simulink model "c28x_spi_eeprom"  (R2021b)
settings: Solver=FixedStepDiscrete  StartTime=0.0  StopTime=Inf  FixedStep=0.001  RelTol=1e-3  EnableMultiTasking=on
libraries: c280xlib x4, svdutilitieslib x2, simulink x2, demo_controls x1
settings Model: SimulationMode=external  ExtModeTrigDuration=8  Creator=The MathWorks, Inc.  LastModifiedBy=The MathWorks, Inc.
settings SolverCC: AlgebraicLoopSolver=TrustRegion
settings DataIOCC: ReturnWorkspaceOutputs=off
settings OptimizationCC: DefaultUnderspecifiedDataType=single  EnhancedBackFolding=on  StrengthReduction=on  PassReuseOutputArgsAs=Individual arguments  MaxStackSize=512  OptimizeBlockOrder=speed  DifferentSizesBufferReuse=on  EfficientTunableParamExpr=on
settings DebuggingCC: InheritedTsInSrcMsg=none  ParameterPrecisionLossMsg=none  ParameterTunabilityLossMsg=error  SFMachineParentedDataDiag=warning  ArithmeticOperatorsInVariantConditions=warning
settings HardwareCC: ProdBitPerChar=16  ProdBitPerInt=16  ProdBitPerPointer=32  ProdBitPerSizeT=32  ProdBitPerPtrDiffT=32  ProdLargestAtomicInteger=Integer  ProdLargestAtomicFloat=None  ProdWordSize=16  ProdLongLongMode=on  ProdHWDeviceType=Texas Instruments->C2000
settings SFSimCC: SimUseLocalCustomCode=off  MATLABDynamicMemAlloc=off  CustomCodeUndefinedFunction=UseInterfaceOnly
settings RTWCC: Description=Embedded Coder  SystemTargetFile=ert.tlc  HardwareBoard=TI Delfino F28379D LaunchPad  TemplateMakefile=ert_default_tmf  GenerateReport=on  RTWUseLocalCustomCode=off  Toolchain=Texas Instruments Code Composer Studio (C2000)  IncludeHyperlinkInReport=on  LaunchReport=on  GenerateTraceInfo=on  GenerateTraceReport=on  GenerateTraceReportSl=on  GenerateTraceReportSf=on  GenerateTraceReportEml=on
settings CodeAppCC: ForceParamTrailComments=on  IgnoreCustomStorageClasses=off  OperatorAnnotations=on  SimulinkDataObjDesc=on  SFDataObjDesc=on  InsertBlockDesc=on
settings ERTTargetCC: CodeReplacementLibrary=TI C28x  ExtModeTransport=4  ExtModeStaticAlloc=on  ExtModeStaticAllocSize=10000  ExtModeMexFile=ext_xcp  ExtModeIntrfLevel=Level2 - Open

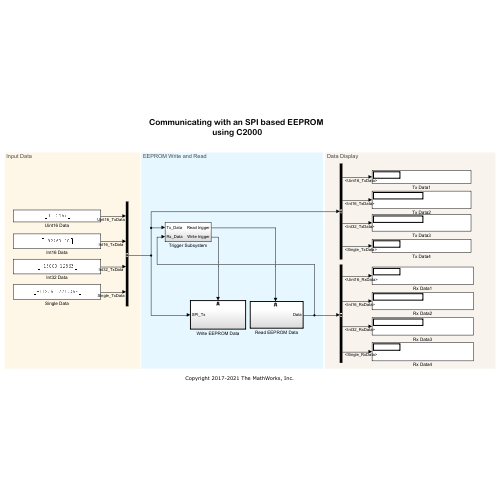
[thumbnail: Simulink's stored preview of the top-level diagram]
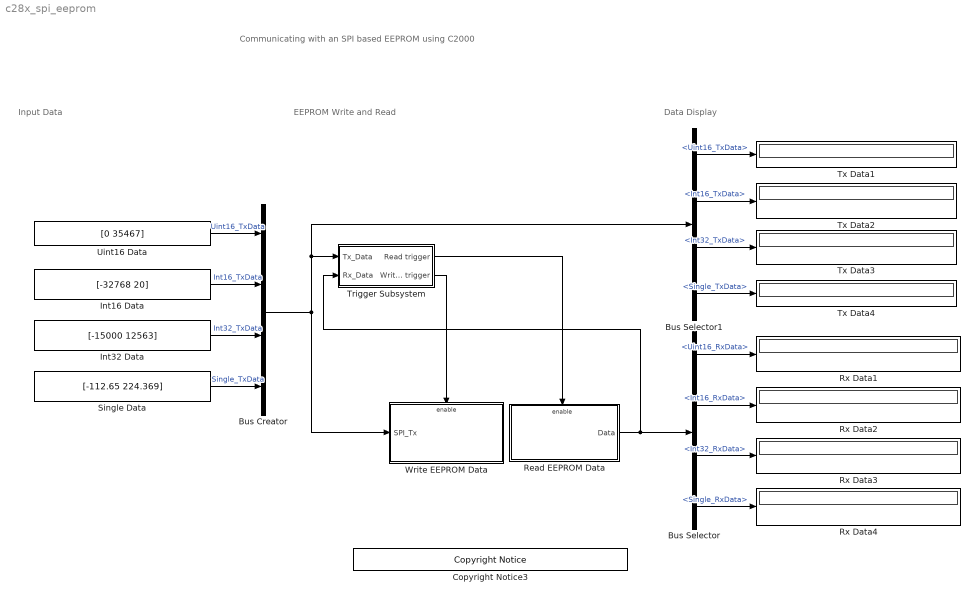
== system c28x_spi_eeprom ==
  note: Communicating with an SPI based EEPROM
      | using C2000
  note: Input Data
  note: EEPROM Write and Read
  note: Data Display
  Bus Creator : BusCreator  Inputs=4
  Bus Selector : BusSelector  OutputSignals=Uint16_RxData,Int16_RxData,Int32_RxData,Single_RxData
  Bus Selector1 : BusSelector  OutputSignals=Uint16_TxData,Int16_TxData,Int32_TxData,Single_TxData
  Copyright Notice3 : demo_controls/Copyright Notice  year=2017  prod=tic2000
      settings: SourceProductBaseCode=ME
  Int16 Data : Constant  Value=[-32768 20]  OutDataTypeStr=int16  SampleTime=-1
  Int32 Data : Constant  Value=[-15000 12563]  OutDataTypeStr=int32  SampleTime=-1
  Read EEPROM Data : Subsystem  TreatAsAtomicUnit=on
  Rx Data{1..4} (4 alike) : Display
      Rx Data4 settings: Format=short_e
  Single Data : Constant  Value=[-112.65 224.369]  OutDataTypeStr=single  SampleTime=-1
  Trigger Subsystem : Subsystem
  Tx Data{1..4} (4 alike) : Display
      Tx Data4 settings: Format=short_e
  Uint16 Data : Constant  Value=[0 35467]  OutDataTypeStr=uint16  SampleTime=-1
  Write EEPROM Data : Subsystem
  wires:
  Trigger Subsystem/1(Read trigger) -> Read EEPROM Data/Enable
  Bus Creator/1 -> Bus Selector1/1, Trigger Subsystem/1(Tx_Data), Write EEPROM Data/1(SPI_Tx)
  Read EEPROM Data/1(Data) -> Trigger Subsystem/2(Rx_Data), Bus Selector/1
  Trigger Subsystem/2(Write trigger) -> Write EEPROM Data/Enable
  Uint16 Data/1 -> Bus Creator/1  "Uint16_TxData"
  Int16 Data/1 -> Bus Creator/2  "Int16_TxData"
  Int32 Data/1 -> Bus Creator/3  "Int32_TxData"
  Single Data/1 -> Bus Creator/4  "Single_TxData"
  Bus Selector/1 -> Rx Data1/1  "<Uint16_RxData>"
  Bus Selector/2 -> Rx Data2/1  "<Int16_RxData>"
  Bus Selector/3 -> Rx Data3/1  "<Int32_RxData>"
  Bus Selector/4 -> Rx Data4/1  "<Single_RxData>"
  Bus Selector1/1 -> Tx Data1/1  "<Uint16_TxData>"
  Bus Selector1/2 -> Tx Data2/1  "<Int16_TxData>"
  Bus Selector1/3 -> Tx Data3/1  "<Int32_TxData>"
  Bus Selector1/4 -> Tx Data4/1  "<Single_TxData>"

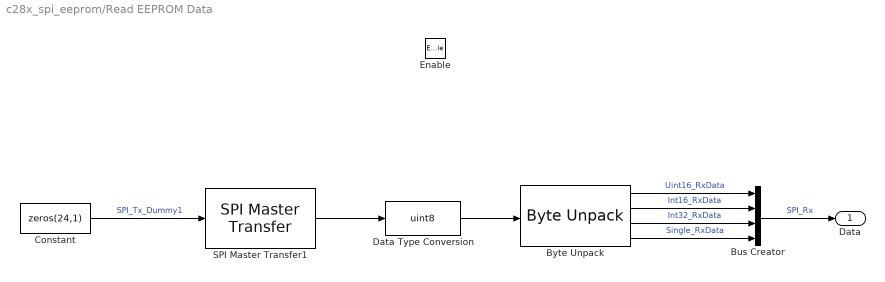
== system c28x_spi_eeprom/Read EEPROM Data ==
  Enable : EnablePort
  Bus Creator : BusCreator  Inputs=4
  Byte Unpack : svdutilitieslib/Byte Unpack  dimensions={2,2,2,2}  datatypes={'uint16','int16','int32','single'}  byteAlign=1  blockPlatform=arduinoert
      settings: SourceProductBaseCode=ANDROID,ARDUINO,ML_ARDUINO,ECCORTEXA,ECCORTEXR,SC_BEAGLEBONE_BLUE,EC_FREEDOM_BOARD,EC_FRDM_K64F,INTEL_BLOCKSET,MICROBIT,NUCLEO,NVIDIA,PX4AUTOPILOTS,RASPPIIO,STMICRODIS,TIC2000,XILINX_BLOCKSET
  Constant : Constant  Value=zeros(24,1)  OutDataTypeStr=uint16
  Data Type Conversion : DataTypeConversion  OutDataTypeStr=uint8
  SPI Master Transfer1 : c280xlib/SPI Master Transfer  SPISelect=SPI_A  ClockPolarity=Rising_edge  ClockPhase=Delay_half_cycle  SPIModule=uint32(0)  Mode=Master  BusSpeed=uint32(1000000)  FirstBitToTransfer=Most significant bit (MSB)  ClockMode=0  BlockFunction=Transfer  EnableRegisterAddress=on  RegisterAddress=[3 0 32]  OutputDataType=int8  OutputDataLength=1  DataBits=8  UseCustomSSPin=Explicit GPIO calls  ActiveLowSSPin=Active low  Pin=1
      settings: SourceProductBaseCode=TIC2000
  Data : Outport  InitialOutput=0  VectorParamsAs1DForOutWhenUnconnected=off
  wires:
  SPI Master Transfer1/1 -> Data Type Conversion/1
  Constant/1 -> SPI Master Transfer1/1  "SPI_Tx_Dummy1"
  Byte Unpack/1 -> Bus Creator/1  "Uint16_RxData"
  Byte Unpack/2 -> Bus Creator/2  "Int16_RxData"
  Byte Unpack/3 -> Bus Creator/3  "Int32_RxData"
  Byte Unpack/4 -> Bus Creator/4  "Single_RxData"
  Bus Creator/1 -> Data/1  "SPI_Rx"
  Data Type Conversion/1 -> Byte Unpack/1

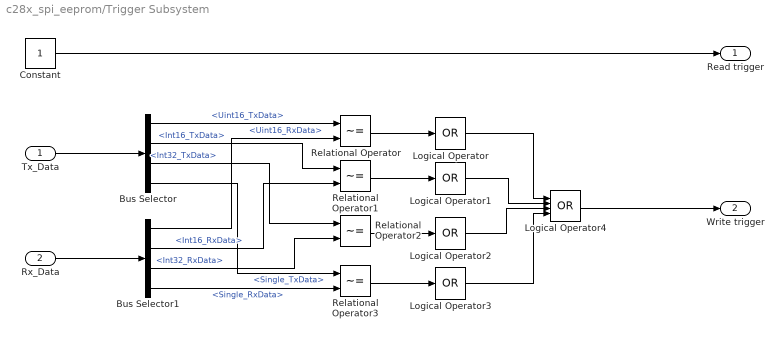
== system c28x_spi_eeprom/Trigger Subsystem ==
  Tx_Data : Inport
  Rx_Data : Inport  Port=2
  Bus Selector : BusSelector  OutputSignals=Uint16_TxData,Int16_TxData,Int32_TxData,Single_TxData
  Bus Selector1 : BusSelector  OutputSignals=Uint16_RxData,Int16_RxData,Int32_RxData,Single_RxData
  Constant : Constant  OutDataTypeStr=uint16  SampleTime=-1
  Logical Operator{,1..3} (4 alike) : Logic  Operator=OR  Inputs=1  AllPortsSameDT=off  OutDataTypeStr=boolean
  Logical Operator4 : Logic  Operator=OR  Inputs=4  AllPortsSameDT=off  OutDataTypeStr=boolean
  Relational Operator{,1..3} (4 alike) : RelationalOperator  Operator=~=  OutDataTypeStr=boolean  RndMeth=Simplest
  Read trigger : Outport  VectorParamsAs1DForOutWhenUnconnected=off
  Write trigger : Outport  Port=2  VectorParamsAs1DForOutWhenUnconnected=off
  wires:
  Constant/1 -> Read trigger/1
  Relational Operator/1 -> Logical Operator/1
  Tx_Data/1 -> Bus Selector/1
  Rx_Data/1 -> Bus Selector1/1
  Relational Operator1/1 -> Logical Operator1/1
  Relational Operator2/1 -> Logical Operator2/1
  Relational Operator3/1 -> Logical Operator3/1
  Bus Selector/1 -> Relational Operator/1  "<Uint16_TxData>"
  Bus Selector1/1 -> Relational Operator/2  "<Uint16_RxData>"
  Bus Selector/2 -> Relational Operator1/1  "<Int16_TxData>"
  Bus Selector1/2 -> Relational Operator1/2  "<Int16_RxData>"
  Bus Selector/3 -> Relational Operator2/1  "<Int32_TxData>"
  Bus Selector1/3 -> Relational Operator2/2  "<Int32_RxData>"
  Bus Selector/4 -> Relational Operator3/1  "<Single_TxData>"
  Logical Operator/1 -> Logical Operator4/1
  Logical Operator1/1 -> Logical Operator4/2
  Logical Operator2/1 -> Logical Operator4/3
  Logical Operator3/1 -> Logical Operator4/4
  Logical Operator4/1 -> Write trigger/1
  Bus Selector1/4 -> Relational Operator3/2  "<Single_RxData>"

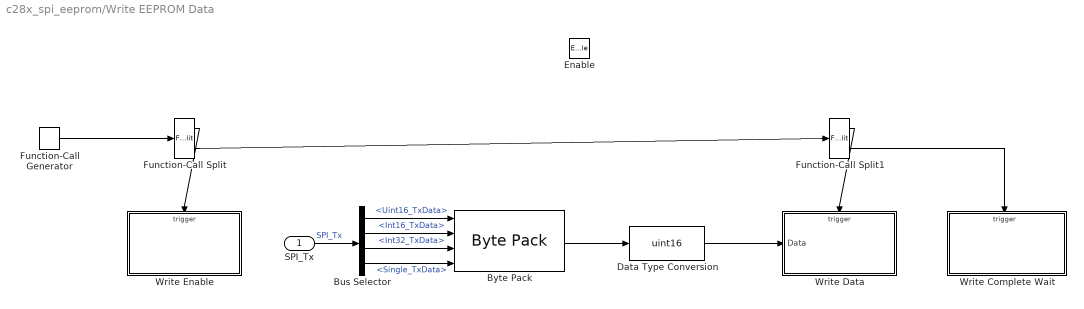
== system c28x_spi_eeprom/Write EEPROM Data ==
  SPI_Tx : Inport
  Enable : EnablePort
  Bus Selector : BusSelector  OutputSignals=Uint16_TxData,Int16_TxData,Int32_TxData,Single_TxData
  Byte Pack : svdutilitieslib/Byte Pack  maskPackedDataType=uint8  datatypes={'uint16','int16','int32','single'}  byteAlign=1  blockPlatform=arduinoert
      settings: SourceProductBaseCode=ANDROID,ARDUINO,ML_ARDUINO,ECCORTEXA,ECCORTEXR,SC_BEAGLEBONE_BLUE,EC_FREEDOM_BOARD,EC_FRDM_K64F,INTEL_BLOCKSET,MICROBIT,NUCLEO,NVIDIA,PX4AUTOPILOTS,RASPPIIO,STMICRODIS,TIC2000,XILINX_BLOCKSET
  Data Type Conversion : DataTypeConversion  OutDataTypeStr=uint16
  Function-Call Generator : simulink/Ports & Subsystems/Function-Call Generator  sample_time=-1  numberOfIterations=1  DisallowWideOutput=off
  Function-Call Split : FunctionCallSplit  NumOutputPorts=2
  Function-Call Split1 : FunctionCallSplit  NumOutputPorts=2
  Write Complete Wait : Subsystem
  Write Data : Subsystem
  Write Enable : Subsystem
  wires:
  Function-Call Generator/1 -> Function-Call Split/1
  Function-Call Split/1 -> Write Enable/Trigger
  Function-Call Split1/2 -> Write Complete Wait/Trigger
  Function-Call Split1/1 -> Write Data/Trigger
  Function-Call Split/2 -> Function-Call Split1/1
  Byte Pack/1 -> Data Type Conversion/1
  SPI_Tx/1 -> Bus Selector/1  "SPI_Tx"
  Data Type Conversion/1 -> Write Data/1(Data)
  Bus Selector/3 -> Byte Pack/3  "<Int32_TxData>"
  Bus Selector/4 -> Byte Pack/4  "<Single_TxData>"
  Bus Selector/1 -> Byte Pack/1  "<Uint16_TxData>"
  Bus Selector/2 -> Byte Pack/2  "<Int16_TxData>"

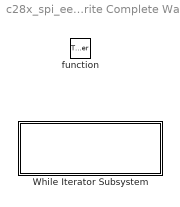
== system c28x_spi_eeprom/Write EEPROM Data/Write Complete Wait ==
  function : TriggerPort  TriggerType=function-call  VariantControl=Variant
  While Iterator Subsystem : Subsystem  Priority=2  TreatAsAtomicUnit=on

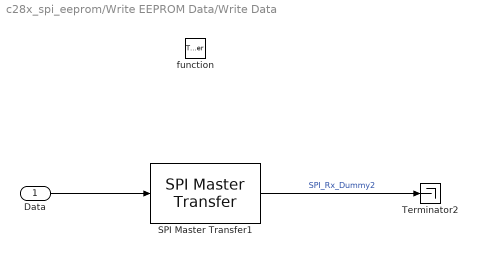
== system c28x_spi_eeprom/Write EEPROM Data/Write Data ==
  Data : Inport
  function : TriggerPort  TriggerType=function-call  VariantControl=Variant
  SPI Master Transfer1 : c280xlib/SPI Master Transfer  SPISelect=SPI_A  ClockPolarity=Rising_edge  ClockPhase=Delay_half_cycle  SPIModule=uint32(0)  Mode=Master  BusSpeed=uint32(1000000)  FirstBitToTransfer=Most significant bit (MSB)  ClockMode=0  BlockFunction=Transfer  EnableRegisterAddress=on  RegisterAddress=[2 0 32]  OutputDataType=int8  OutputDataLength=1  DataBits=8  UseCustomSSPin=Explicit GPIO calls  ActiveLowSSPin=Active low  Pin=1
      settings: SourceProductBaseCode=TIC2000
  Terminator2 : Terminator
  wires:
  SPI Master Transfer1/1 -> Terminator2/1  "SPI_Rx_Dummy2"
  Data/1 -> SPI Master Transfer1/1

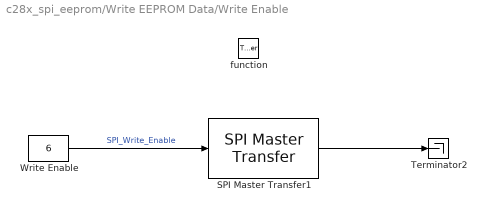
== system c28x_spi_eeprom/Write EEPROM Data/Write Enable ==
  function : TriggerPort  TriggerType=function-call  VariantControl=Variant
  SPI Master Transfer1 : c280xlib/SPI Master Transfer  SPISelect=SPI_A  ClockPolarity=Rising_edge  ClockPhase=Delay_half_cycle  SPIModule=uint32(0)  Mode=Master  BusSpeed=uint32(1000000)  FirstBitToTransfer=Most significant bit (MSB)  ClockMode=0  BlockFunction=Transfer  EnableRegisterAddress=off  RegisterAddress=0  OutputDataType=int8  OutputDataLength=1  DataBits=8  UseCustomSSPin=Explicit GPIO calls  ActiveLowSSPin=Active low  Pin=1
      settings: SourceProductBaseCode=TIC2000
  Terminator2 : Terminator
  Write Enable : Constant  Value=6  OutDataTypeStr=uint16  SampleTime=-1
  wires:
  SPI Master Transfer1/1 -> Terminator2/1
  Write Enable/1 -> SPI Master Transfer1/1  "SPI_Write_Enable"

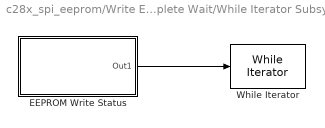
== system c28x_spi_eeprom/Write EEPROM Data/Write Complete Wait/While Iterator Subsystem ==
  EEPROM Write Status : Subsystem
  While Iterator : WhileIterator  MaxIters=-1  WhileBlockType=do-while
  wires:
  EEPROM Write Status/1(Out1) -> While Iterator/1

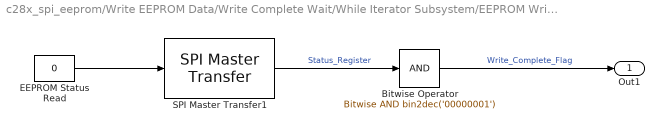
== system c28x_spi_eeprom/Write EEPROM Data/Write Complete Wait/While Iterator Subsystem/EEPROM Write Status ==
  Bitwise Operator : simulink/Logic and Bit Operations/Bitwise Operator  logicop=AND  UseBitMask=on  BitMask=bin2dec('00000001')  BitMaskRealWorld=Stored Integer
  EEPROM Status Read : Constant  Value=0  OutDataTypeStr=uint16  SampleTime=-1
  SPI Master Transfer1 : c280xlib/SPI Master Transfer  SPISelect=SPI_A  ClockPolarity=Rising_edge  ClockPhase=Delay_half_cycle  SPIModule=uint32(0)  Mode=Master  BusSpeed=uint32(1000000)  FirstBitToTransfer=Most significant bit (MSB)  ClockMode=0  BlockFunction=Transfer  EnableRegisterAddress=on  RegisterAddress=5  OutputDataType=int8  OutputDataLength=1  DataBits=8  UseCustomSSPin=Explicit GPIO calls  ActiveLowSSPin=Active low  Pin=1
      settings: SourceProductBaseCode=TIC2000
  Out1 : Outport  VectorParamsAs1DForOutWhenUnconnected=off
  wires:
  EEPROM Status Read/1 -> SPI Master Transfer1/1
  Bitwise Operator/1 -> Out1/1  "Write_Complete_Flag"
  SPI Master Transfer1/1 -> Bitwise Operator/1  "Status_Register"
